simulink model "Simulacao"  (R2013b)
settings: Solver=ode45  StartTime=0.0  StopTime=10.0  RelTol=1e-3
settings Model: Creator=Eduardo  LastModifiedBy=Eduardo
settings OptimizationCC: OptimizeModelRefInitCode=on  LifeSpan=1
settings RTWCC: SystemTargetFile=ert.tlc  TemplateMakefile=ert_default_tmf  Description=Embedded Coder  GenerateReport=on  ProcessScript=ert_make_rtw_hook  IncludeHyperlinkInReport=on  LaunchReport=on  GenerateTraceInfo=on  GenerateTraceReport=on  GenerateTraceReportSl=on  GenerateTraceReportSf=on  GenerateTraceReportEml=on
settings CodeAppCC: IgnoreCustomStorageClasses=off
settings ERTTargetCC: CodeReplacementLibrary=ANSI_C  GenerateSampleERTMain=on  ERTCustomFileTemplate=example_file_process.tlc

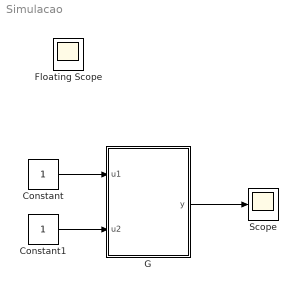
== system Simulacao ==
  Constant : Constant  OutDataTypeStr=int32
  Constant1 : Constant  OutDataTypeStr=int32
  G : Subsystem
  Scope : Scope
  Floating Scope : Scope
      settings: Floating=on
  wires:
  Constant/1 -> G/1(u1)
  Constant1/1 -> G/2(u2)
  G/1(y) -> Scope/1

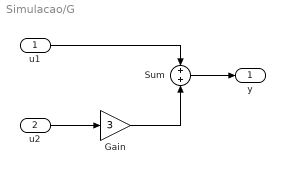
== system Simulacao/G ==
  u1 : Inport  OutDataTypeStr=int32
  u2 : Inport  Port=2  OutDataTypeStr=int32
  Gain : Gain  Gain=3  ParamDataTypeStr=int32  OutDataTypeStr=int32
  Sum : Sum  Inputs=+|+
  y : Outport  OutDataTypeStr=int32
  wires:
  u1/1 -> Sum/1
  Gain/1 -> Sum/2
  u2/1 -> Gain/1
  Sum/1 -> y/1
